simulink model "Fault_Analyzer_Example_FaultModel_3"  (R2025b)
settings: Solver=VariableStepAuto  StartTime=0.0  StopTime=10.0  RelTol=1e-3  EnableMultiTasking=on
settings Model: Creator=georg  LastModifiedBy=georg
settings DebuggingCC: InheritedTsInSrcMsg=none

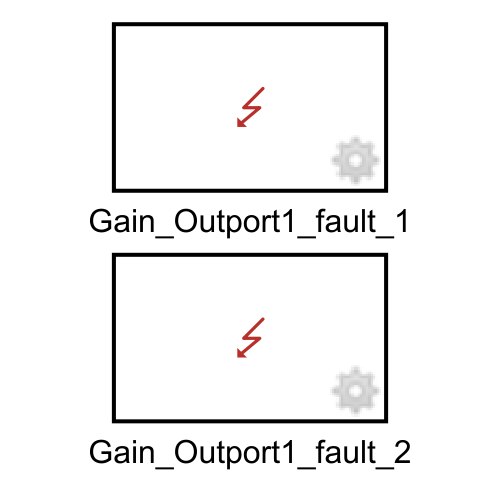
[thumbnail: Simulink's stored preview of the top-level diagram]
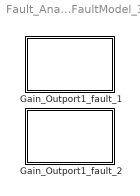
== system Fault_Analyzer_Example_FaultModel_3 ==
  Gain_Outport1_fault_1 : Subsystem  TreatAsAtomicUnit=on  IsInjectorSS=on
  Gain_Outport1_fault_2 : Subsystem  TreatAsAtomicUnit=on  IsInjectorSS=on

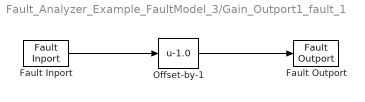
== system Fault_Analyzer_Example_FaultModel_3/Gain_Outport1_fault_1 ==
  Fault Inport : FaultInport
  Fault Outport : FaultOutport
  Offset-by-1 : Bias  Bias=-1.0  SaturateOnIntegerOverflow=off
  wires:
  Fault Inport/1 -> Offset-by-1/1
  Offset-by-1/1 -> Fault Outport/1

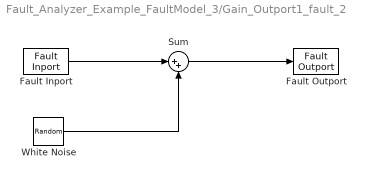
== system Fault_Analyzer_Example_FaultModel_3/Gain_Outport1_fault_2 ==
  Fault Inport : FaultInport
  Fault Outport : FaultOutport
  Sum : Sum  Inputs=|++  OutDataTypeStr=Inherit: Inherit via back propagation
  White Noise : RandomNumber  DisableCoverage=on  Seed=[23341]
  wires:
  White Noise/1 -> Sum/2
  Sum/1 -> Fault Outport/1
  Fault Inport/1 -> Sum/1
